simulink model "tc_from_ctf"  (R2024a)
settings: Solver=VariableStepAuto  StartTime=0.0  StopTime=10  RelTol=1e-3
values from neighbouring files (symbols this model uses):
  user_input = input(promt)    [temperature_conversion_from_C_to_F.m]
settings Model: Creator=admin  LastModifiedBy=admin

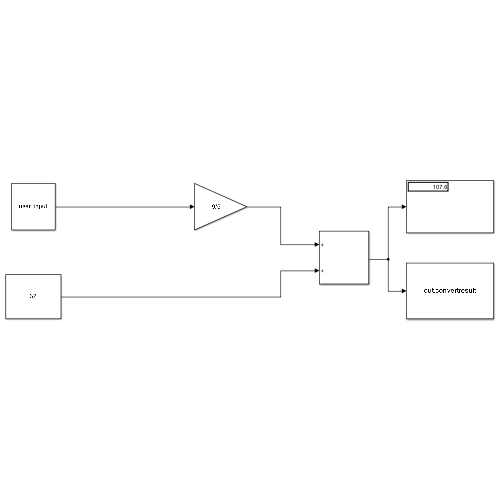
[thumbnail: Simulink's stored preview of the top-level diagram]
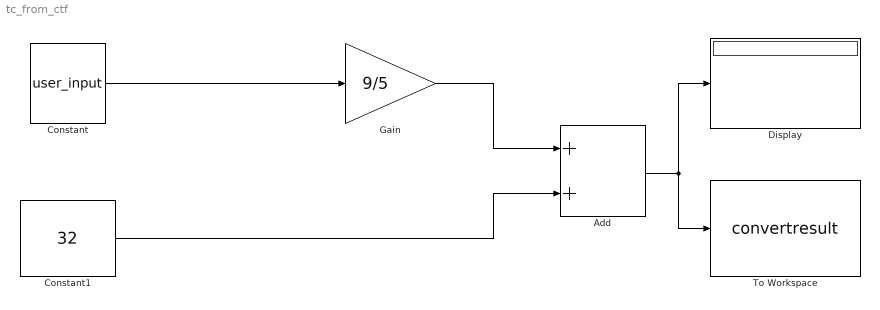
== system tc_from_ctf ==
  Add : Sum
  Constant : Constant  Value=user_input
  Constant1 : Constant  Value=32
  Display : Display
  Gain : Gain  Gain=9/5
  To Workspace : ToWorkspace  VariableName=convertresult  SaveFormat=Timeseries  SampleTime=-1
  wires:
  Constant/1 -> Gain/1
  Constant1/1 -> Add/2
  Gain/1 -> Add/1
  Add/1 -> To Workspace/1, Display/1
